simulink model "FUZZPID"  (R2016a)
settings: Solver=VariableStepAuto  StartTime=0.0  StopTime=5.0  RelTol=1e-3
libraries: fuzblock x1
settings Model: Creator=Li Yingping  LastModifiedBy=Li Yingping

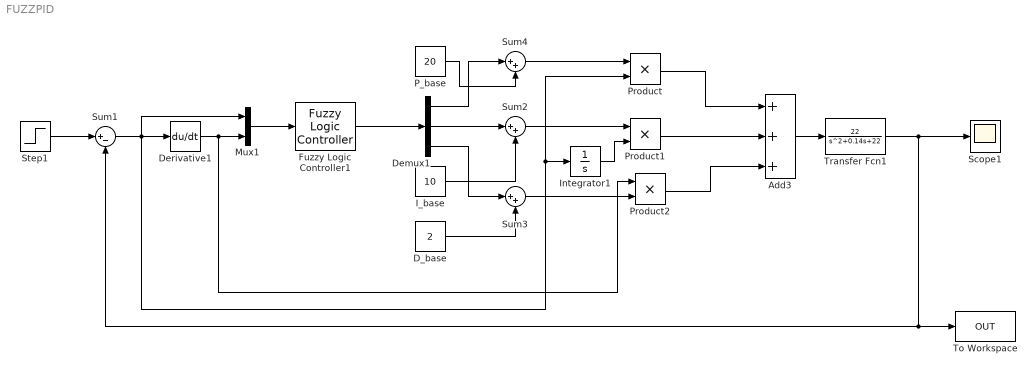
== system FUZZPID ==
  Add3 : Sum  Inputs=+++
  D_base : Constant  Value=2
  Demux1 : Demux  Outputs=3
  Derivative1 : Derivative
  Fuzzy Logic Controller1 : fuzblock/Fuzzy Logic  Controller  fis=fuzzpid
  I_base : Constant  Value=10
  Integrator1 : Integrator
  Mux1 : Mux  Inputs=2
  P_base : Constant  Value=20
  Product : Product  RndMeth=Zero
  Product1 : Product  RndMeth=Zero
  Product2 : Product  RndMeth=Zero
  Scope1 : Scope
  Step1 : Step  Time=0  SampleTime=0
  Sum1 : Sum  Inputs=|+-
  Sum2 : Sum  Inputs=|++
  Sum3 : Sum  Inputs=|++
  Sum4 : Sum  Inputs=|++
  To Workspace : ToWorkspace  VariableName=OUT  SaveFormat=Timeseries  SampleTime=-1
  Transfer Fcn1 : TransferFcn  Numerator=[22]  Denominator=[1 0.14 22]
  wires:
  Step1/1 -> Sum1/1
  Sum1/1 -> Mux1/1, Product/2, Integrator1/1, Derivative1/1
  Transfer Fcn1/1 -> Scope1/1, To Workspace/1, Sum1/2
  Derivative1/1 -> Product2/1, Mux1/2
  Mux1/1 -> Fuzzy Logic Controller1/1
  Fuzzy Logic Controller1/1 -> Demux1/1
  Demux1/3 -> Sum3/1
  Demux1/2 -> Sum2/1
  Demux1/1 -> Sum4/1
  P_base/1 -> Sum4/2
  I_base/1 -> Sum2/2
  D_base/1 -> Sum3/2
  Product2/1 -> Add3/3
  Product/1 -> Add3/1
  Integrator1/1 -> Product1/2
  Product1/1 -> Add3/2
  Add3/1 -> Transfer Fcn1/1
  Sum3/1 -> Product2/2
  Sum2/1 -> Product1/1
  Sum4/1 -> Product/1
